simulink model "Sanboks_SIMULINK_v0_3_R2020a"  (R2020a)
settings: Solver=ode45  StartTime=0  StopTime=1600  FixedStep=1  RelTol=1e-4
undefined symbols (not defined in the file): achievable_velocity, air_density, car_mass, coefficient_rolling_resistance, conti_PID, conti_rpm, conti_torque, current, distance, drag_coefficient, final_drivetrain_efficiency, front_braking_torque, frontal_area, gear_ratio, grade_of_track, gravity, no_laps, no_of_motors, peak_PID, peak_rpm, peak_torque, Rear_braking_torque, reference_steering_angle, rot_mass, start_time_for_peak, steering_ratio, supply_voltage, tire_radius, track_length, x_leng
libraries: simulink x4
settings Model: Creator=Swapnil Mane  LastModifiedBy=rk
settings SolverCC: MaxConsecutiveMinStep=auto  ZeroCrossAlgorithm=Adaptive  SolverResetMethod=Robust
settings DebuggingCC: AlgebraicLoopMsg=none  MaskedZcDiagnostic=none  IgnoredZcDiagnostic=none

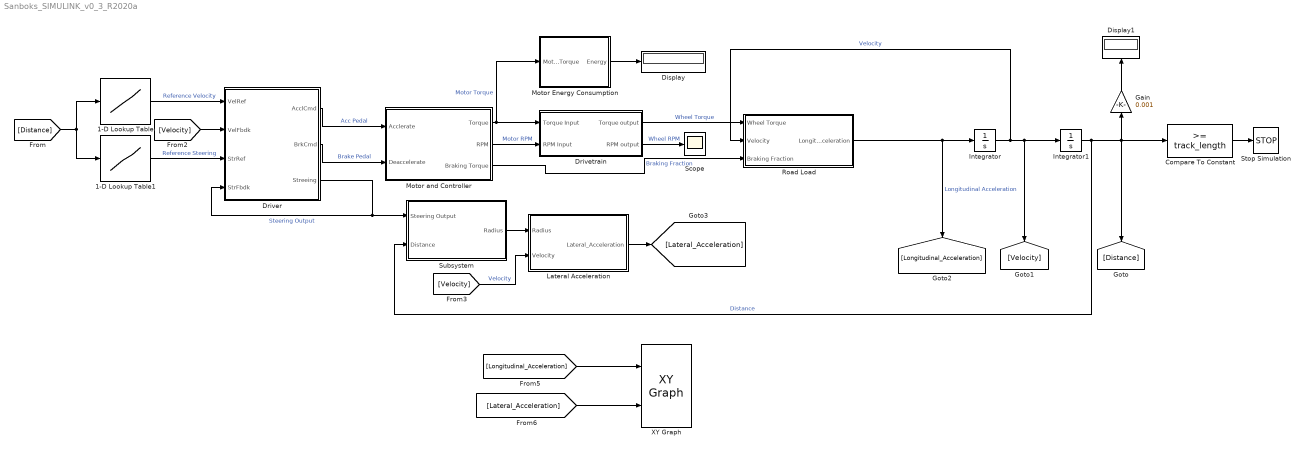
== system Sanboks_SIMULINK_v0_3_R2020a ==
  1-D Lookup Table : Lookup_n-D  NumberOfTableDimensions=1  BreakpointsForDimension1=distance(1:2:x_leng*no_laps)  Table=achievable_velocity  InternalRulePriority=Speed  RndMeth=Simplest  InputSameDT=on
  1-D Lookup Table1 : Lookup_n-D  NumberOfTableDimensions=1  BreakpointsForDimension1=distance(1:x_leng*no_laps)  Table=reference_steering_angle  InternalRulePriority=Speed  RndMeth=Simplest  InputSameDT=on
  Compare To Constant : simulink/Logic and Bit Operations/Compare To Constant  relop=>=  const=track_length  OutDataTypeStr=boolean
  Display : Display
  Display1 : Display
  Driver : Subsystem
      mask Display: image('$imagefile'); % Use "Edit Image" on toolstrip to change.
  Drivetrain : Subsystem
      mask Display: image('$imagefile'); % Use "Edit Image" on toolstrip to change.
  Gain : Gain  Gain=0.001
  Integrator : Integrator
  Integrator1 : Integrator
  Lateral Acceleration : Subsystem
  Motor Energy Consumption : Subsystem
  Motor and Controller : Subsystem
      mask Display: image('$imagefile'); % Use "Edit Image" on toolstrip to change.
  Road Load : Subsystem
  Scope : Scope
  Stop Simulation : Stop
  Subsystem : Subsystem
  XY Graph : simulink/Sinks/XY Graph  xmin=-20  xmax=20  ymin=-20  ymax=20  st=-1
  wires:
  Driver/1(AcclCmd) -> Motor and Controller/1(Acclerate)  "Acc Pedal"
  Motor and Controller/1(Torque) -> Drivetrain/1(Torque Input), Motor Energy Consumption/1(Motor Torque)  "Motor Torque"
  Motor and Controller/2(" RPM") -> Drivetrain/2(RPM Input)  "Motor RPM"
  Driver/2(BrkCmd) -> Motor and Controller/2(Deaccelerate)  "Brake Pedal"
  Compare To Constant/1 -> Stop Simulation/1
  Integrator1/1 -> Compare To Constant/1, Gain/1, [Distance], Subsystem/2(Distance)  "Distance"
  1-D Lookup Table/1 -> Driver/1(VelRef)  "Reference Velocity"
  Integrator/1 -> Integrator1/1, [Velocity], Road Load/2(Velocity)  "Velocity"
  1-D Lookup Table1/1 -> Driver/3(StrRef)  "Reference Steering"
  Driver/3(Streeing) -> Driver/4(StrFbdk), Subsystem/1(Steering Output)  "Steering Output"
  [Velocity] -> Driver/2(VelFbdk)
  [Velocity] -> Lateral Acceleration/2(Velocity)  "Velocity"
  Lateral Acceleration/1(Lateral_Acceleration) -> [Lateral_Acceleration]
  [Lateral_Acceleration] -> XY Graph/2
  [Longitudinal_Acceleration] -> XY Graph/1
  Subsystem/1(Radius) -> Lateral Acceleration/1(Radius)
  Motor Energy Consumption/1(Energy) -> Display/1
  Drivetrain/2(RPM output) -> Scope/1  "Wheel RPM"
  [Distance] -> 1-D Lookup Table1/1, 1-D Lookup Table/1
  Road Load/1(Longitunal Acceleration) -> [Longitudinal_Acceleration], Integrator/1  "Longitudinal Acceleration"
  Drivetrain/1(Torque output) -> Road Load/1(Wheel Torque)  "Wheel Torque"
  Motor and Controller/3(Braking Torque) -> Road Load/3(Braking Fraction)  "Braking Fraction"
  Gain/1 -> Display1/1

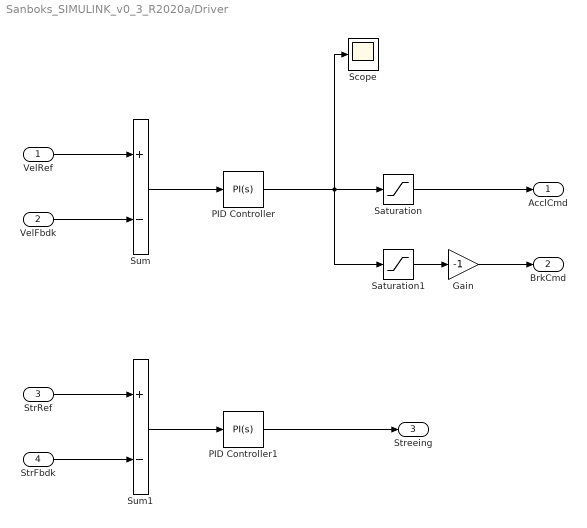
== system Sanboks_SIMULINK_v0_3_R2020a/Driver ==
  VelRef : Inport
  VelFbdk : Inport  Port=2
  StrRef : Inport  Port=3
  StrFbdk : Inport  Port=4
  Gain : Gain  Gain=-1
  PID Controller : simulink/Continuous/PID Controller  Controller=PI  Form=Parallel  TimeDomain=Continuous-time  UseExternalTs=off  SampleTime=-1  IntegratorMethod=Forward Euler  FilterMethod=Forward Euler  ControllerParametersSource=internal  P=1  I=0  D=0  UseFilter=on  N=10  TunerSelectOption=Transfer Function Based (PID Tuner App)  InitialConditionSource=internal  InitialConditionForIntegrator=0  InitialConditionForFilter=0  DifferentiatorICPrevScaledInput=0  ExternalReset=none  TrackingMode=off  Kt=1  LimitOutput=off  UpperSaturationLimit=inf  LowerSaturationLimit=-inf  LinearizeAsGain=on  AntiWindupMode=none  Kb=1  POutMin=[]  POutMax=[]  IOutMin=[]  IOutMax=[]  DOutMin=[]  DOutMax=[]  NOutMin=[]  NOutMax=[]  SumOutMin=[]  SumOutMax=[]  SaturationOutMin=[]  SaturationOutMax=[]  PParamMin=[]  PParamMax=[]  IParamMin=[]  IParamMax=[]  DParamMin=[]  DParamMax=[]  NParamMin=[]  NParamMax=[]  KbParamMin=[]  KbParamMax=[]  KtParamMin=[]  KtParamMax=[]  KbOutMin=[]  KbOutMax=[]  KtOutMin=[]  KtOutMax=[]  IntegratorOutMin=[]  IntegratorOutMax=[]  FilterOutMin=[]  FilterOutMax=[]  SumI1OutMin=[]  SumI1OutMax=[]  SumI2OutMin=[]  SumI2OutMax=[]  SumI3OutMin=[]  SumI3OutMax=[]  SumI4OutMin=[]  SumI4OutMax=[]  SumDOutMin=[]  SumDOutMax=[]  DifferentiatorOutMin=[]  DifferentiatorOutMax=[]  FilterDiffOutCoefMin=[]  FilterDiffOutCoefMax=[]  ReciprocalOutMin=[]  ReciprocalOutMax=[]  SumDenOutMin=[]  SumDenOutMax=[]  SumNumOutMin=[]  SumNumOutMax=[]  DivideOutMin=[]  DivideOutMax=[]  UdiffTsProdOutMin=[]  UdiffTsProdOutMax=[]  NTsProdOutMin=[]  NTsProdOutMax=[]  UintegralTsProdOutMin=[]  UintegralTsProdOutMax=[]  UngainTsProdOutMin=[]  UngainTsProdOutMax=[]  IntegratorContinuousStateAttributes=''  IntegratorStateMustResolveToSignalObject=off  IntegratorRTWStateStorageClass=Auto  FilterContinuousStateAttributes=''  FilterStateMustResolveToSignalObject=off  FilterRTWStateStorageClass=Auto  ParallelPVariant=InternalParameters  IdealPVariant=Disabled  IVariant=InternalParameters  DVariant=Disabled  IntegratorVariant=Continuous  SatVariant=Disabled  AWVariant=Passthrough  PCopyVariant=Disabled  TRVariant=Disabled  FdbkBlocksVariant=Forward  IdealPFdbkVariant=Disabled  SatFdbkVariant=Disabled  DerivativeFilterVariant=Disabled  NVariant=Disabled  NCopyVariant=Disabled_SignalSpec  FilterICVariant=Disabled  IntegratorICVariant=InternalICs  ExternalResetVariant=Disabled  TRSumVariant=Passthrough  SumFdbkVariant=Disabled  SumVariant=Sum_PI  TsampFilterVariant=InternalTs  TsampNgainVariant=Passthrough  TsampIntegralVariant=Passthrough
  PID Controller1 : simulink/Continuous/PID Controller  Controller=PI  Form=Parallel  TimeDomain=Continuous-time  UseExternalTs=off  SampleTime=-1  IntegratorMethod=Forward Euler  FilterMethod=Forward Euler  ControllerParametersSource=internal  P=1  I=0  D=0  UseFilter=on  N=10  TunerSelectOption=Transfer Function Based (PID Tuner App)  InitialConditionSource=internal  InitialConditionForIntegrator=0  InitialConditionForFilter=0  DifferentiatorICPrevScaledInput=0  ExternalReset=none  TrackingMode=off  Kt=1  LimitOutput=off  UpperSaturationLimit=inf  LowerSaturationLimit=-inf  LinearizeAsGain=on  AntiWindupMode=none  Kb=1  POutMin=[]  POutMax=[]  IOutMin=[]  IOutMax=[]  DOutMin=[]  DOutMax=[]  NOutMin=[]  NOutMax=[]  SumOutMin=[]  SumOutMax=[]  SaturationOutMin=[]  SaturationOutMax=[]  PParamMin=[]  PParamMax=[]  IParamMin=[]  IParamMax=[]  DParamMin=[]  DParamMax=[]  NParamMin=[]  NParamMax=[]  KbParamMin=[]  KbParamMax=[]  KtParamMin=[]  KtParamMax=[]  KbOutMin=[]  KbOutMax=[]  KtOutMin=[]  KtOutMax=[]  IntegratorOutMin=[]  IntegratorOutMax=[]  FilterOutMin=[]  FilterOutMax=[]  SumI1OutMin=[]  SumI1OutMax=[]  SumI2OutMin=[]  SumI2OutMax=[]  SumI3OutMin=[]  SumI3OutMax=[]  SumI4OutMin=[]  SumI4OutMax=[]  SumDOutMin=[]  SumDOutMax=[]  DifferentiatorOutMin=[]  DifferentiatorOutMax=[]  FilterDiffOutCoefMin=[]  FilterDiffOutCoefMax=[]  ReciprocalOutMin=[]  ReciprocalOutMax=[]  SumDenOutMin=[]  SumDenOutMax=[]  SumNumOutMin=[]  SumNumOutMax=[]  DivideOutMin=[]  DivideOutMax=[]  UdiffTsProdOutMin=[]  UdiffTsProdOutMax=[]  NTsProdOutMin=[]  NTsProdOutMax=[]  UintegralTsProdOutMin=[]  UintegralTsProdOutMax=[]  UngainTsProdOutMin=[]  UngainTsProdOutMax=[]  IntegratorContinuousStateAttributes=''  IntegratorStateMustResolveToSignalObject=off  IntegratorRTWStateStorageClass=Auto  FilterContinuousStateAttributes=''  FilterStateMustResolveToSignalObject=off  FilterRTWStateStorageClass=Auto  ParallelPVariant=InternalParameters  IdealPVariant=Disabled  IVariant=InternalParameters  DVariant=Disabled  IntegratorVariant=Continuous  SatVariant=Disabled  AWVariant=Passthrough  PCopyVariant=Disabled  TRVariant=Disabled  FdbkBlocksVariant=Forward  IdealPFdbkVariant=Disabled  SatFdbkVariant=Disabled  DerivativeFilterVariant=Disabled  NVariant=Disabled  NCopyVariant=Disabled_SignalSpec  FilterICVariant=Disabled  IntegratorICVariant=InternalICs  ExternalResetVariant=Disabled  TRSumVariant=Passthrough  SumFdbkVariant=Disabled  SumVariant=Sum_PI  TsampFilterVariant=InternalTs  TsampNgainVariant=Passthrough  TsampIntegralVariant=Passthrough
  Saturation : Saturate  UpperLimit=1  LowerLimit=0
  Saturation1 : Saturate  UpperLimit=0  LowerLimit=-1
  Scope : Scope
  Sum : Sum  Inputs=+-
  Sum1 : Sum  Inputs=+-
  AcclCmd : Outport
  BrkCmd : Outport  Port=2
  Streeing : Outport  Port=3
  wires:
  PID Controller/1 -> Saturation1/1, Saturation/1, Scope/1
  VelFbdk/1 -> Sum/2
  Sum/1 -> PID Controller/1
  VelRef/1 -> Sum/1
  Saturation/1 -> AcclCmd/1
  Gain/1 -> BrkCmd/1
  Saturation1/1 -> Gain/1
  StrRef/1 -> Sum1/1
  Sum1/1 -> PID Controller1/1
  StrFbdk/1 -> Sum1/2
  PID Controller1/1 -> Streeing/1

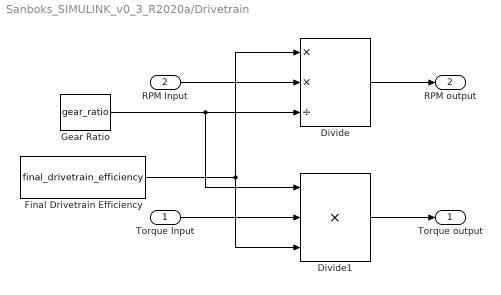
== system Sanboks_SIMULINK_v0_3_R2020a/Drivetrain ==
  Torque Input : Inport
  RPM Input : Inport  Port=2
  Divide : Product  Inputs=**/
  Divide1 : Product  Inputs=***
  Final Drivetrain Efficiency : Constant  Value=final_drivetrain_efficiency
  Gear Ratio : Constant  Value=gear_ratio
  Torque output : Outport
  RPM output : Outport  Port=2
  wires:
  Gear Ratio/1 -> Divide/3, Divide1/1
  Final Drivetrain Efficiency/1 -> Divide1/3, Divide/1
  RPM Input/1 -> Divide/2
  Divide/1 -> RPM output/1
  Torque Input/1 -> Divide1/2
  Divide1/1 -> Torque output/1

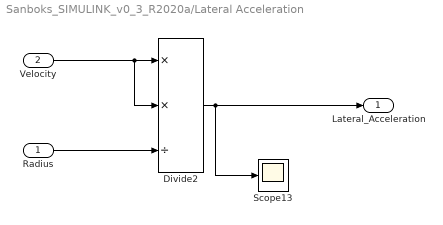
== system Sanboks_SIMULINK_v0_3_R2020a/Lateral Acceleration ==
  Radius : Inport
  Velocity : Inport  Port=2
  Divide2 : Product  Inputs=**/
  Scope13 : Scope
  Lateral_Acceleration : Outport
  wires:
  Divide2/1 -> Lateral_Acceleration/1, Scope13/1
  Radius/1 -> Divide2/3
  Velocity/1 -> Divide2/2, Divide2/1

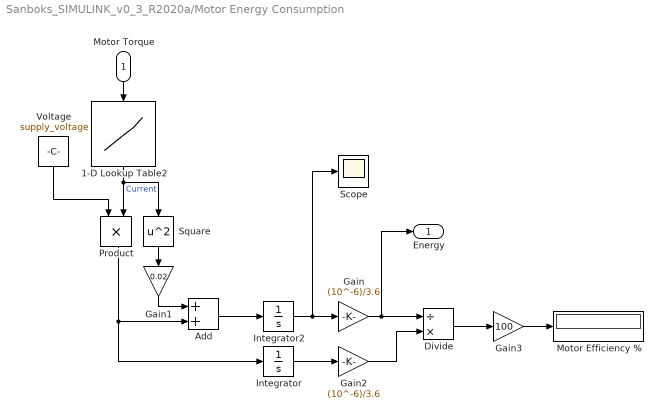
== system Sanboks_SIMULINK_v0_3_R2020a/Motor Energy Consumption ==
  Motor Torque : Inport
  1-D Lookup Table2 : Lookup_n-D  NumberOfTableDimensions=1  BreakpointsForDimension1=peak_torque  Table=current  InternalRulePriority=Speed  RndMeth=Simplest  InputSameDT=on
  Add : Sum
  Divide : Product  Inputs=/*
  Gain : Gain  Gain=(10^-6)/3.6
  Gain1 : Gain  Gain=0.02
  Gain2 : Gain  Gain=(10^-6)/3.6
  Gain3 : Gain  Gain=100
  Integrator : Integrator
  Integrator2 : Integrator
  Motor Efficiency % : Display
  Product : Product
  Scope : Scope
  Square : Math  Operator=square  SaturateOnIntegerOverflow=on
  Voltage : Constant  Value=supply_voltage
  Energy : Outport
  wires:
  Product/1 -> Integrator/1, Add/2
  Gain1/1 -> Add/1
  Voltage/1 -> Product/1
  Add/1 -> Integrator2/1
  1-D Lookup Table2/1 -> Product/2, Square/1  "Current"
  Integrator2/1 -> Scope/1, Gain/1
  Motor Torque/1 -> 1-D Lookup Table2/1
  Gain/1 -> Energy/1, Divide/1
  Square/1 -> Gain1/1
  Integrator/1 -> Gain2/1
  Gain2/1 -> Divide/2
  Divide/1 -> Gain3/1
  Gain3/1 -> Motor Efficiency %/1

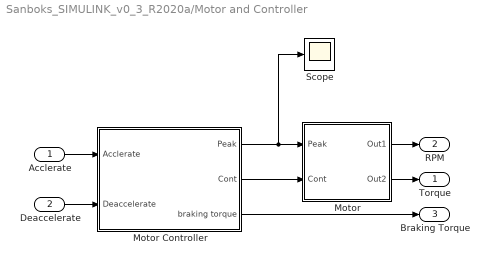
== system Sanboks_SIMULINK_v0_3_R2020a/Motor and Controller ==
  Acclerate : Inport
  Deaccelerate : Inport  Port=2
  Motor : Subsystem
  Motor Controller : Subsystem
  Scope : Scope
  Torque : Outport
  " RPM" : Outport  Port=2
  Braking Torque : Outport  Port=3
  wires:
  Acclerate/1 -> Motor Controller/1(Acclerate)
  Deaccelerate/1 -> Motor Controller/2(Deaccelerate)
  Motor Controller/1(Peak) -> Scope/1, Motor/1(Peak)
  Motor Controller/2(Cont) -> Motor/2(Cont)
  Motor/1(Out1) -> " RPM"/1
  Motor/2(Out2) -> Torque/1
  Motor Controller/3(braking torque) -> Braking Torque/1

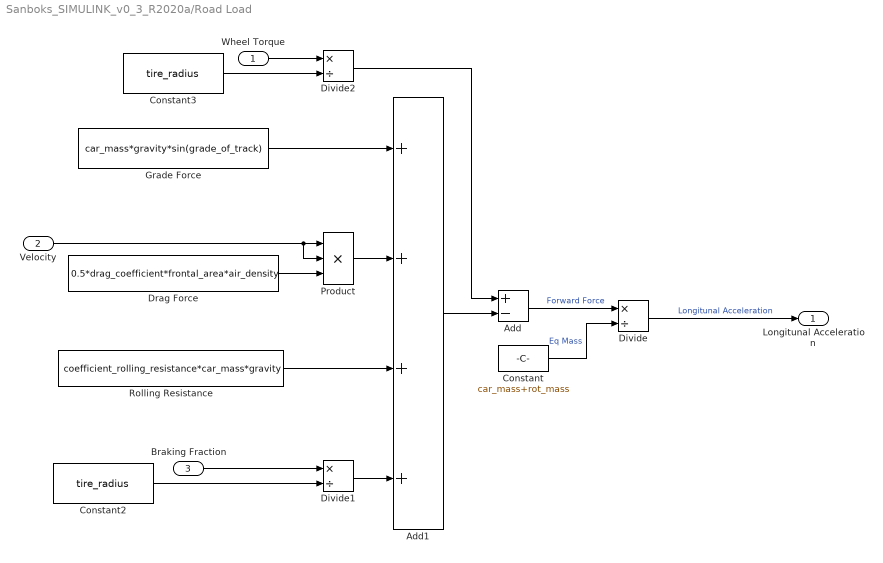
== system Sanboks_SIMULINK_v0_3_R2020a/Road Load ==
  Wheel Torque : Inport
  Velocity : Inport  Port=2
  Braking Fraction : Inport  Port=3
  Add : Sum  Inputs=+-
  Add1 : Sum  Inputs=++++
  Constant : Constant  Value=car_mass+rot_mass
  Constant2 : Constant  Value=tire_radius
  Constant3 : Constant  Value=tire_radius
  Divide : Product  Inputs=*/
  Divide1 : Product  Inputs=*/
  Divide2 : Product  Inputs=*/
  Drag Force : Constant  Value=0.5*drag_coefficient*frontal_area*air_density
  Grade Force : Constant  Value=car_mass*gravity*sin(grade_of_track)
  Product : Product  Inputs=3
  Rolling Resistance : Constant  Value=coefficient_rolling_resistance*car_mass*gravity
  Longitunal Acceleration : Outport
  wires:
  Product/1 -> Add1/2
  Grade Force/1 -> Add1/1
  Add1/1 -> Add/2
  Drag Force/1 -> Product/3
  Constant/1 -> Divide/2  "Eq Mass"
  Braking Fraction/1 -> Divide1/1
  Add/1 -> Divide/1  "Forward Force"
  Constant2/1 -> Divide1/2
  Divide1/1 -> Add1/4
  Rolling Resistance/1 -> Add1/3
  Constant3/1 -> Divide2/2
  Divide2/1 -> Add/1
  Velocity/1 -> Product/2, Product/1
  Divide/1 -> Longitunal Acceleration/1  "Longitunal Acceleration"
  Wheel Torque/1 -> Divide2/1

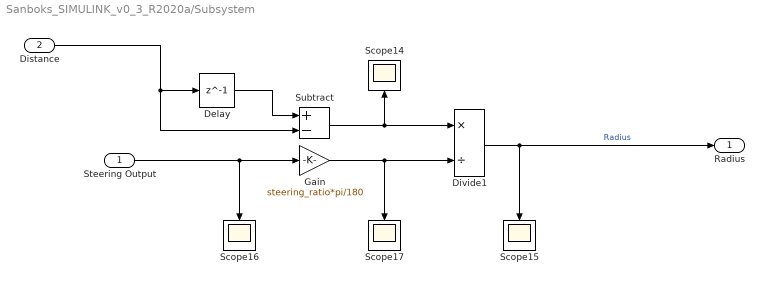
== system Sanboks_SIMULINK_v0_3_R2020a/Subsystem ==
  Steering Output : Inport
  Distance : Inport  Port=2
  Delay : Delay  DelayLength=1
  Divide1 : Product  Inputs=*/
  Gain : Gain  Gain=steering_ratio*pi/180
  Scope{14..17} (4 alike) : Scope
  Subtract : Sum  Inputs=+-
  Radius : Outport
  wires:
  Distance/1 -> Subtract/2, Delay/1
  Gain/1 -> Divide1/2, Scope17/1
  Subtract/1 -> Divide1/1, Scope14/1
  Divide1/1 -> Scope15/1, Radius/1  "Radius"
  Steering Output/1 -> Scope16/1, Gain/1
  Delay/1 -> Subtract/1

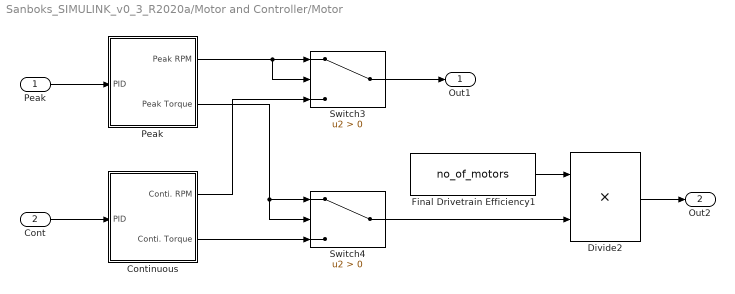
== system Sanboks_SIMULINK_v0_3_R2020a/Motor and Controller/Motor ==
  Peak : Inport
  Cont : Inport  Port=2
  Continuous : Subsystem
  Divide2 : Product  Inputs=**
  Final Drivetrain Efficiency1 : Constant  Value=no_of_motors
  "Peak " : Subsystem
  Switch3 : Switch  Criteria=u2 > Threshold
  Switch4 : Switch  Criteria=u2 > Threshold
  Out1 : Outport
  Out2 : Outport  Port=2
  wires:
  Cont/1 -> Continuous/1(PID)
  "Peak "/2(Peak Torque) -> Switch4/2, Switch4/1
  "Peak "/1(Peak RPM) -> Switch3/2, Switch3/1
  Continuous/1(Conti. RPM) -> Switch3/3
  Switch3/1 -> Out1/1
  Peak/1 -> "Peak "/1(PID)
  Continuous/2(Conti. Torque) -> Switch4/3
  Switch4/1 -> Divide2/2
  Final Drivetrain Efficiency1/1 -> Divide2/1
  Divide2/1 -> Out2/1

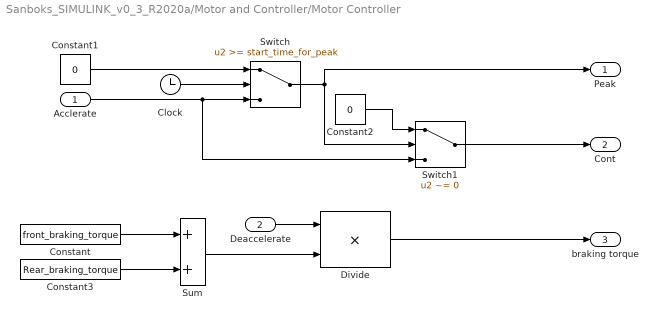
== system Sanboks_SIMULINK_v0_3_R2020a/Motor and Controller/Motor Controller ==
  Acclerate : Inport
  Deaccelerate : Inport  Port=2
  Clock : Clock
  Constant : Constant  Value=front_braking_torque
  Constant1 : Constant  Value=0
  Constant2 : Constant  Value=0
  Constant3 : Constant  Value=Rear_braking_torque
  Divide : Product  Inputs=**
  Sum : Sum
  Switch : Switch  Threshold=start_time_for_peak
  Switch1 : Switch  Criteria=u2 ~= 0
  Peak : Outport
  Cont : Outport  Port=2
  braking torque : Outport  Port=3
  wires:
  Acclerate/1 -> Switch/3, Switch1/3
  Switch/1 -> Peak/1, Switch1/2
  Switch1/1 -> Cont/1
  Deaccelerate/1 -> Divide/1
  Divide/1 -> braking torque/1
  Constant3/1 -> Sum/2
  Constant/1 -> Sum/1
  Sum/1 -> Divide/2
  Clock/1 -> Switch/2
  Constant1/1 -> Switch/1
  Constant2/1 -> Switch1/1

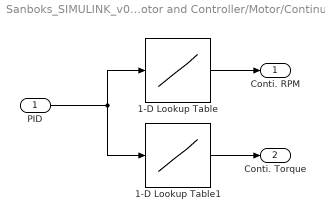
== system Sanboks_SIMULINK_v0_3_R2020a/Motor and Controller/Motor/Continuous ==
  PID : Inport
  1-D Lookup Table : Lookup_n-D  NumberOfTableDimensions=1  BreakpointsForDimension1=conti_PID  Table=conti_rpm  InternalRulePriority=Speed  RndMeth=Simplest  InputSameDT=on
  1-D Lookup Table1 : Lookup_n-D  NumberOfTableDimensions=1  BreakpointsForDimension1=conti_PID  Table=conti_torque  InternalRulePriority=Speed  RndMeth=Simplest  InputSameDT=on
  Conti. RPM : Outport
  Conti. Torque : Outport  Port=2
  wires:
  1-D Lookup Table/1 -> Conti. RPM/1
  PID/1 -> 1-D Lookup Table1/1, 1-D Lookup Table/1
  1-D Lookup Table1/1 -> Conti. Torque/1

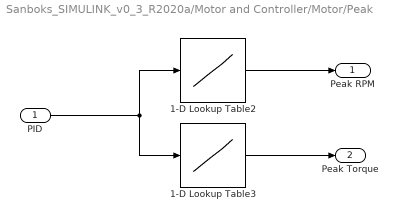
== system Sanboks_SIMULINK_v0_3_R2020a/Motor and Controller/Motor/Peak  ==
  PID : Inport
  1-D Lookup Table2 : Lookup_n-D  NumberOfTableDimensions=1  BreakpointsForDimension1=peak_PID  Table=peak_rpm  InternalRulePriority=Speed  RndMeth=Simplest  InputSameDT=on
  1-D Lookup Table3 : Lookup_n-D  NumberOfTableDimensions=1  BreakpointsForDimension1=peak_PID  Table=peak_torque  InternalRulePriority=Speed  RndMeth=Simplest  InputSameDT=on
  Peak RPM : Outport
  Peak Torque : Outport  Port=2
  wires:
  PID/1 -> 1-D Lookup Table3/1, 1-D Lookup Table2/1
  1-D Lookup Table2/1 -> Peak RPM/1
  1-D Lookup Table3/1 -> Peak Torque/1
